simulink model "MPC_Constraint"  (Simulink 10.2)
settings: Solver=FixedStepDiscrete  StartTime=0.0  StopTime=8  FixedStep=0.001  RelTol=1e-3
libraries: simulink x4, Solver_SF x1
settings Model: Creator=TINNER  LastModifiedBy=TINNER
settings DataIOCC: SaveFormat=Dataset  SignalLoggingSaveFormat=Dataset
settings OptimizationCC: LifeSpan=auto
settings DebuggingCC: UnderspecifiedInitializationDetection=Simplified  MergeDetectMultiDrivingBlocksExec=error  FcnCallInpInsideContextMsg=error  SFUnexpectedBacktrackingDiag=error  SFNoUnconditionalDefaultTransitionDiag=error  SFExecutionAtInitializationDiag=warning  ArithmeticOperatorsInVariantConditions=error
settings HardwareCC: ProdBitPerPointer=64  ProdBitPerSizeT=64  ProdBitPerPtrDiffT=64  ProdLargestAtomicFloat=Float  ProdIntDivRoundTo=Zero  ProdEndianess=LittleEndian  ProdWordSize=64  ProdHWDeviceType=Intel->x86-64 (Windows64)
settings ModelReferenceCC: PropagateSignalLabelsOutOfModel=on
settings SFSimCC: SimUseLocalCustomCode=on  CustomCodeUndefinedFunction=FilterOut
settings RTWCC: RTWUseLocalCustomCode=on
settings CodeAppCC: StateflowObjectComments=off
settings GRTTargetCC: TargetLangStandard=C99 (ISO)  CombineOutputUpdateFcns=on  GRTInterface=off
settings ConfigComp: CovMetricSettings=dwe  CovSaveCumulativeToWorkspaceVar=off  CovSaveSingleToWorkspaceVar=off  CovExternalEMLEnable=on

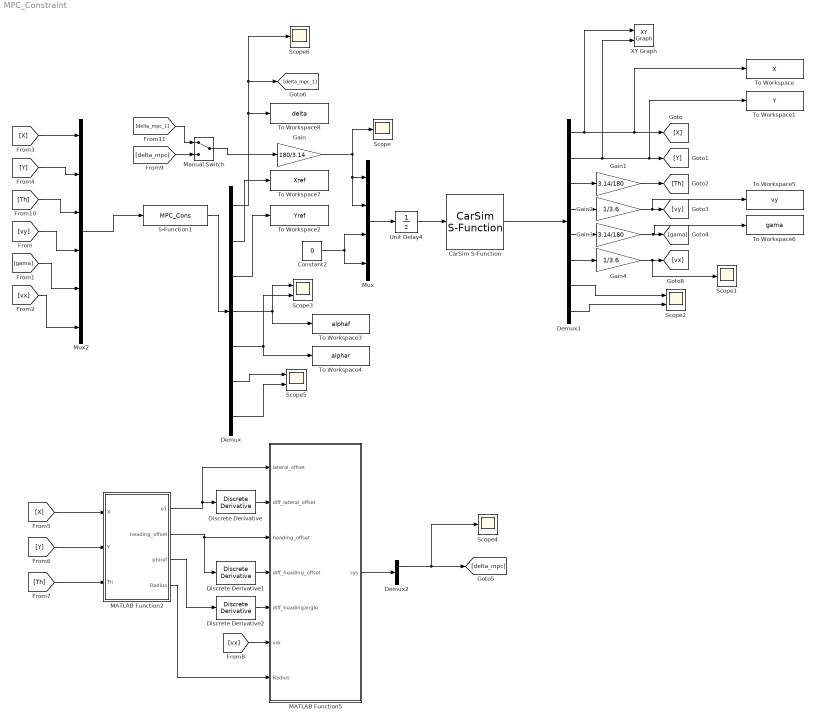
== system MPC_Constraint ==
  CarSim S-Function : Solver_SF/CarSim S-Function  Priority=1  SIMFILE=simfile.sim  Run_RTs=off  vs_state_ind=Run  StopMode_ind=Vehicle Model
  Constant2 : Constant  Value=0
  Demux : Demux  Outputs=7
  Demux1 : Demux  Outputs=8
  Demux2 : Demux  Outputs=2
  Discrete Derivative : simulink/Discrete/Discrete Derivative  gainval=1.0  ICPrevScaledInput=0.0  OutMin=[]  OutMax=[]  OutDataType=fixdt(1, 16)  OutScaling=2^-10  DoSatur=off
  Discrete Derivative1 : simulink/Discrete/Discrete Derivative  gainval=1.0  ICPrevScaledInput=0.0  OutMin=[]  OutMax=[]  OutDataType=fixdt(1, 16)  OutScaling=2^-10  DoSatur=off
  Discrete Derivative2 : simulink/Discrete/Discrete Derivative  gainval=1.0  ICPrevScaledInput=0.0  OutMin=[]  OutMax=[]  OutDataType=fixdt(1, 16)  OutScaling=2^-10  DoSatur=off
  Gain : Gain  Gain=180/3.14
  Gain1 : Gain  Gain=3.14/180
  Gain2 : Gain  Gain=1/3.6
  Gain3 : Gain  Gain=3.14/180
  Gain4 : Gain  Gain=1/3.6
  MATLAB Function2 : MATLAB Function  TreatAsAtomicUnit=on
  MATLAB Function5 : MATLAB Function  TreatAsAtomicUnit=on
  Manual Switch : ManualSwitch
  Mux : Mux
  Mux2 : Mux  Inputs=6
  S-Function1 : S-Function  FunctionName=MPC_Cons  SFunctionDeploymentMode=off  EnableBusSupport=off
  Scope{,1,4,6} (4 alike) : Scope
  Scope2 : Scope  NumInputPorts=2
  Scope3 : Scope  NumInputPorts=2
  Scope5 : Scope  NumInputPorts=2
  To Workspace : ToWorkspace  VariableName=X  SampleTime=-1
  To Workspace1 : ToWorkspace  VariableName=Y  SampleTime=-1
  To Workspace2 : ToWorkspace  VariableName=Yref  SampleTime=-1
  To Workspace3 : ToWorkspace  VariableName=alphaf  SampleTime=-1
  To Workspace4 : ToWorkspace  VariableName=alphar  SampleTime=-1
  To Workspace5 : ToWorkspace  VariableName=vy  SampleTime=-1
  To Workspace6 : ToWorkspace  VariableName=gama  SampleTime=-1
  To Workspace7 : ToWorkspace  VariableName=Xref  SampleTime=-1
  To Workspace8 : ToWorkspace  VariableName=delta  SampleTime=-1
  Unit Delay4 : UnitDelay  SampleTime=-1  HasFrameUpgradeWarning=on
  XY Graph : simulink/Sinks/XY Graph  xmin=-1  xmax=200  ymin=-10  ymax=10  st=-1
  wires:
  Demux1/1 -> XY Graph/1, To Workspace/1, [X]
  Demux1/2 -> XY Graph/2, To Workspace1/1, [Y]
  Mux/1 -> Unit Delay4/1
  Gain/1 -> Mux/2, Mux/1, Scope/1
  Constant2/1 -> Mux/4, Mux/3
  Gain1/1 -> [Th]
  Demux1/3 -> Gain1/1
  Gain2/1 -> To Workspace5/1, [vy]
  Demux1/4 -> Gain2/1
  Demux1/5 -> Gain3/1
  Gain3/1 -> To Workspace6/1, [gama]
  Gain4/1 -> Scope1/1, [vx]
  Demux1/6 -> Gain4/1
  S-Function1/1 -> Demux/1
  Demux/1 -> To Workspace8/1, Scope6/1, [delta_mpc_1]
  Demux1/7 -> Scope2/1
  Demux1/8 -> Scope2/2
  CarSim S-Function/1 -> Demux1/1
  [X] -> Mux2/1
  [Y] -> Mux2/2
  Mux2/1 -> S-Function1/1
  [vx] -> Mux2/6
  [gama] -> Mux2/5
  [vy] -> Mux2/4
  [Th] -> Mux2/3
  Unit Delay4/1 -> CarSim S-Function/1
  Demux/5 -> Scope3/2, To Workspace4/1
  Demux/4 -> Scope3/1, To Workspace3/1
  Demux/3 -> To Workspace2/1
  Demux/2 -> To Workspace7/1
  MATLAB Function2/1(e1) -> Discrete Derivative/1, MATLAB Function5/1(lateral_offset)
  Discrete Derivative/1 -> MATLAB Function5/2(diff_lateral_offset)
  MATLAB Function2/2(heading_offset) -> Discrete Derivative1/1, MATLAB Function5/3(heading_offset)
  Discrete Derivative1/1 -> MATLAB Function5/4(diff_heading_offset)
  [X] -> MATLAB Function2/1(X)
  [Y] -> MATLAB Function2/2(Y)
  [Th] -> MATLAB Function2/3(Th)
  Discrete Derivative2/1 -> MATLAB Function5/5(diff_headingangle)
  MATLAB Function2/3(phiref) -> Discrete Derivative2/1
  [vx] -> MATLAB Function5/6(vdr)
  MATLAB Function2/4(Radius) -> MATLAB Function5/7(Radius)
  MATLAB Function5/1(sys) -> Demux2/1
  Demux2/1 -> Scope4/1, [delta_mpc]
  [delta_mpc] -> Manual Switch/2
  Manual Switch/1 -> Gain/1
  [delta_mpc_1] -> Manual Switch/1
  Demux/6 -> Scope5/1
  Demux/7 -> Scope5/2

== matlab function MATLAB Function2 ==
  data: e1 output double; X input double; Y input double; Th input double; heading_offset output double; phiref output double; Radius output double
function [e1,heading_offset,phiref, Radius] = fcn(X,Y,Th)
% A_trans = [cos(Thr) sin(Thr);
%            -sin(Thr) cos(Thr)];
% x = zeros(2,1);
% x = A_trans*[X-Xr;Y-Yr];
% e1 = x(2);
% 
% heading_offset = Th - Thr;
% if (heading_offset < -pi)
%     heading_offset = heading_offset + 2*pi;
% end
% if (heading_offset > pi)
%     heading_offset = heading_offset - 2*pi;
% end
Dp = 5;
[eymin,ephi,phiref,Yref]=ref(X,Y,Th,Dp)
e1=-eymin;
heading_offset=-ephi;
K=curvature(X);
Radius=1/K;
 function [eymin,ephi,phiref,Yref]=ref(X,Y,phi,Dp)
        Xt=X+Dp*cos(phi);
        Yt=Y+Dp*sin(phi);
        %% 单移线工况预瞄横向偏差参数 %%
%         d=7.6;
%         l=120;
%         Yref=d/(2*pi)*(pi+2*pi*(Xt-l/2)/l+sin(2*pi/l*(Xt-l/2)));
%         phiref=(2723726541130763*pi)/135107988821114880 + (2723726541130763*pi*cos((pi*(Xt - 60))/60))/135107988821114880;
%         if Xt>120
%             Yref = 7.6;
%             phiref = 0;
%         end
        %% 双移线工况预瞄横向偏差参数 %%
            shape=2.4;%参数名称，用于参考轨迹生成
    dx1=25;dx2=21.95;%没有任何实际意义，只是参数名称
    dy1=4.05;dy2=5.7;%没有任何实际意义，只是参数名称
    Xs1=27.19;Xs2=56.46;%参数名称
    z1=shape/dx1*(Xt-Xs1)-shape/2;
    z2=shape/dx2*(Xt-Xs2)-shape/2;
    Yref=dy1/2*(1+tanh(z1))-dy2/2*(1+tanh(z2));
    phiref=atan(dy1*(1/cosh(z1))^2*(1.2/dx1)-dy2*(1/cosh(z2))^2*(1.2/dx2));
        eymin=Yref-Yt;
        ephi=phiref-phi;
 end

        function K=curvature(X)
        %将以下注释输入到命令行窗口，在工作区获得曲率方程
%         syms t;
%         d=7.6;
%         l=120;
%         fx=d/(2*pi)*(pi+2*pi*(t-l/2)/l+sin(2*pi/l*(t-l/2)));%单移线
%         fK=diff(fx,t,2)/(1+diff(fx,t,1)^2)^(3/2);
        %采用论文中的K
%         if  X<=20 || X>=105
%             K=0;
%         else if  X>20 && X<=60
%                 K=5*10^(-3);
%             else
%                 K=-5*10^(-3);
%             end
%         end
%% 单移线K
%         K=-(2723726541130763*pi^2*sin((pi*(X - 60))/60))/(8106479329266892800*(((2723726541130763*pi)/135107988821114880 + (2723726541130763*pi*cos((pi*(X - 60))/60))/135107988821114880)^2 + 1)^(3/2));
%% 双移线K
        K=((243*tanh((12*X)/125 - 11907/3125)*((12*tanh((12*X)/125 - 11907/3125)^2)/125 - 12/125))/625 - (1368*tanh((48*X)/439 - 80922/10975)*((48*tanh((48*X)/439 - 80922/10975)^2)/439 - 48/439))/2195)/(((243*tanh((12*X)/125 - 11907/3125)^2)/1250 - (684*tanh((48*X)/439 - 80922/10975)^2)/2195 + 64323/548750)^2 + 1)^(3/2);
        end

end

== matlab function MATLAB Function5 ==
  data: lateral_offset input double; diff_lateral_offset input double; heading_offset input double; diff_heading_offset input double; diff_headingangle input double; vdr input double; sys output double; Radius input double
function sys = fcn(lateral_offset,diff_lateral_offset,heading_offset,diff_heading_offset,diff_headingangle,vdr,Radius)
persistent U u_piao
if isempty(U)
U = zeros(1,1);
end
if isempty(u_piao)
u_piao = zeros(1,1);
end
if vdr==0
    vdr=5;
end
if Radius<40
    Radius=40;
end
m = 1270;
Iz = 1536.7;
lf = 1.015;
L = 2.910;
lr = L-1.015;
Cf = 46241;
Cr = 66666;
Np = 6;
Nc = 6;
Nx = 4;
Nu = 1;
q1 = 100;
q2 = 0.1;
q3 = 1;
q4 = 0.1;
r1 = 5;
T = 0.01;% 采样时间
a22 = -2*(Cf+Cr)/m/vdr;
a23 = 2*(Cf+Cr)/m;
a24 = -2*(lf*Cf-lr*Cr)/m/vdr;
a42 = -2*(lf*Cf-lr*Cr)/Iz/vdr;
a43 = 2*(lf*Cf-lr*Cr)/Iz;
a44 = -2*(lf^2*Cf+lr^2*Cr)/Iz/vdr;
Am = [0 1 0 0;
      0 a22 a23 a24;
      0 0 0 1;
      0 a42 a43 a44];
A = (eye(4)-Am*T/2)^(-1)*(eye(4)+Am*T/2);
Bm = [0;
      Cf/m;
      0;
      lf*Cf/Iz];
B = Bm*T;
D = [0;
     -(lf*Cf-lr*Cr)/m/vdr-vdr;
     0;
     -(lf^2*Cf+lr^2*Cr)/Iz/vdr];

% diff_lateral_offset = vdr * sin(diff_heading_offset);
% diff_heading_offset = diff_headingangle-vdr*K;
dxk = [lateral_offset;
       diff_lateral_offset;
       heading_offset;
       diff_heading_offset];
   
Q_cell = cell(Np,Np);
    for i = 1:1:Np
        for j = 1:1:Np
            if i == j
                Q_cell{i,j} = [q1 0 0 0;
                               0 q2 0 0;
                               0 0 q3 0;
                               0 0 0 q4];
            else
                Q_cell{i,j} = zeros(Nx,Nx);
            end
        end
    end
    
Q = My_cell2mat(Q_cell);
R = r1*eye(Nu*Nc);

C=[ 1 0 0 0;
    0 1 0 0;
    0 0 1 0;
    0 0 0 1];

PHI_cell = cell(Np,1);
Sb_cell = cell(Np,1);
THETA_cell = cell(Np,Nc);
for j=1:1:Np
    PHI_cell{j,1}=C*A^j;
    if j==1
        Sb_cell{j,1}=C*A^j*D;
    else
        Sb_cell{j,1}=Sb_cell{j-1,1}+C*A^j*D;
    end
    for k=1:1:Nc
        if k<=j
           THETA_cell{j,k}=C*A^(j-k)*B;
        else 
           THETA_cell{j,k}=zeros(Nx,Nu);
        end
    end
end


PHI=My_cell2mat(PHI_cell);%size(PHI)=[Nx*Np Nx+Nu]
THETA=My_cell2mat(THETA_cell);%size(THETA)=[Nx*Np Nu*(Nc+1)]
Sb=My_cell2mat(Sb_cell);
H=THETA'*Q*THETA+R;
H=(H+H')/2;

error=PHI*dxk+Sb*diff_headingangle;
% error=PHI*dxk;
f=2*error'*Q*THETA;

A_t=zeros(Nc,Nc);
for p=1:1:Nc
    for q=1:1:Nc
        if q<=p
            A_t(p,q)=1;
        else
            A_t(p,q)=0;
        end
    end
end
% A_I=kron(A_t,eye(Nu));
A_I=kron([-1;0],eye(Nc));
U = [0 1/vdr 0 lf/vdr;
     0 1/vdr 0 -lf/vdr]*dxk;
Ut=kron(ones(Nc,1), U);
umin=[-0.0523;-0.0523];
umax=[0.0523;0.0523]; 
delta_umin = -0.82; 
delta_umax = 0.82;

Umin=kron(ones(Nc,1),umin);
Umax=kron(ones(Nc,1),umax);
A_cons_cell={A_I zeros(Nu*Nc, 1); -A_I zeros(Nu*Nc, 1)};
b_cons_cell={Umax-Ut;-Umin+Ut};
A_cons=[A_I; -A_I];
b_cons=[Umax-Ut;-Umin+Ut];

   % 状态量约束
delta_Umin = kron(ones(Nc,1),delta_umin);
delta_Umax = kron(ones(Nc,1),delta_umax);
lb = delta_Umin;
ub = delta_Umax;


options = optimoptions('quadprog','Algorithm','active-set');
x_start = zeros(Nu*Nc,1);
[Xout, fval,exitflag]=quadprog(H, f, [], [],[],[],lb,ub,x_start,options);
% [Xout, fval,exitflag]=quadprog(H, f, A_cons, b_cons,[],[],lb,ub,x_start,options);
% u_real = zeros(2,1);
% u_piao(1)=Xout(1); % X1为二次规划求出来的是控制时域内最优的速度控制增量
% u_piao(2)=Xout(2); % X2为二次规划求出来的最优前轮转角控制增量
% U(1)=dxk(4)+u_piao(1); %kesi4为速度误差。kesi4为速度误差与速度误差增量u_piao(1)相加得到我们下一时刻的kesi矩阵的第四行
% U(2)=dxk(5)+u_piao(2); %kesi5为k-1时刻前轮偏角误差，道理同上，与前轮偏角误差的增量相加得到我们下一时刻的kesi矩阵的第五行
% u_real(1)=U(1)+vdr; %再与下面的参考速度相加才是真正的速度
% u_real(2)=U(2)+Deltar; %道理同上
Kv = lr*m/2/Cf/L-lf*m/2/Cr/L;
K3 = 1;
feedforward_steeringangle = L/Radius+Kv*vdr^2/Radius-K3*(lr/Radius-lf*m*vdr^2/Radius/L/2/Cr);
sys = [Xout(1);feedforward_steeringangle];
% sys = [0;0];

% function Matrix=My_cell2mat(u)
% [cell_rows,cell_cols]=size(u);
% sum_rows = 0;
% sum_cols = 0;
% for ii=1:1:cell_rows
%     [rows,cols]=size(u{ii,1});
%     sum_rows=sum_rows+rows;
% end    
% for jj=1:1:cell_cols
%     [rows,cols]=size(u{1,jj});
%     sum_cols=sum_cols+cols;
% end
% Matrix_temp=zeros(sum_rows,sum_cols);
% 
% sum_rows=0;
% for ii=1:1:cell_rows
%     sum_cols=0;
%     for jj=1:1:cell_cols
%         [Row,Col]=size(u{ii,jj});
%         for aa=1:1:Row
%             for bb=1:1:Col
%                 Matrix_temp(sum_rows+aa,sum_cols+bb)=u{ii,jj}(aa,bb);
%             end
%         end
%         sum_cols=sum_cols+Col; 
%     end
%     sum_rows=sum_rows+Row;
% end
% Matrix=Matrix_temp;
% % Matrix=u;
% end


function Matrix=My_cell2mat(u)
[cell_rows,cell_cols]=size(u);
[rows,cols]=size(u{1,1});
Matrix_temp=zeros(cell_rows*rows,cell_cols*cols);
for ii=1:1:cell_rows
    for jj=1:1:cell_cols
        [Row,Col]=size(u{ii,jj});
        for a=1:1:Row
            for b=1:1:Col
                Matrix_temp((ii-1)*Row+a,(jj-1)*Col+b)=u{ii,jj}(a,b);
            end
        end
    end
end
Matrix=Matrix_temp;
end

end
